simulink model "WormAndGearConstraint"  (R2024a)
settings: Solver=ode45  StartTime=0.0  StopTime=120  MaxStep=0.01  RelTol=1e-3
PreLoadFcn:
  | addpath(fullfile('WormAndGearConstraintSupport','Data'));
  | addpath(fullfile('WormAndGearConstraintSupport','Scripts'));
model workspace: external: MATLAB File WormAndGearConstraintParameters.m (data not in the file)
undefined symbols (not defined in the file or in its folder): slewdrive, X, Y, Z
libraries: sm_lib x75, neural x40, nesl_utility x38, fl_lib x32, WormAndGearConstraintLibrary x24, ee_lib x6, slpidlib x6, spsSeriesRLCBranchLib x2, fl_ps_legacy_lib x1, spsPWMGeneratorDCDCLib x1, spsMosfetLib x1, spsPVArrayLib x1
(part 6 of 6)

== system WormAndGearConstraint/Solar Array/Solar Tracker3/Slew Drive/Worm and Gear Assembly/Worm ==
  Left Non-Threaded : WormAndGearConstraintLibrary/Sliced Hollow Cylinder  outerRadius=wormNonThreadedRadius  thickness=wormNonThreadedThickness  length=wormNonThreadedLength  sliceThickness=wormSliceProportion*wormNonThreadedRadius  rho=wormRho  mainColor=wormColor  sliceColor=wormSliceColor
  Right Non-Threaded : WormAndGearConstraintLibrary/Sliced Hollow Cylinder  outerRadius=wormNonThreadedRadius  thickness=wormNonThreadedThickness  length=wormNonThreadedLength  sliceThickness=wormSliceProportion*wormNonThreadedRadius  rho=wormRho  mainColor=wormColor  sliceColor=wormSliceColor
  Threaded : WormAndGearConstraintLibrary/Sliced Hollow Cylinder  outerRadius=wormRadius  thickness=wormThreadedThickness  length=wormThreadedLength  sliceThickness=wormSliceProportion*wormRadius  rho=wormRho  mainColor=wormColor  sliceColor=wormSliceColor
  L : PMIOPort  Side=Left
  R : PMIOPort  Port=2  Side=Right
  connections:
  Threaded/LConn1 -- Left Non-Threaded/RConn1
  Threaded/RConn1 -- Right Non-Threaded/LConn1
  R/RConn1 -- Right Non-Threaded/RConn1
  Left Non-Threaded/LConn1 -- L/RConn1

== matlab function WormAndGearConstraint/Soalr Power Generation Calculation/Solar inputs1/MATLAB Function1 ==
  data: lat input; output output; lon input
function output = generateInput(lat, lon)
    % Get the current date and time
    datetimeNow = datetime('now');
    [~, month, day , hour, ~, ~] = datevec(datetimeNow);

    % Create the output array
    output = [lat; lon; month; day; hour];
end

== matlab function WormAndGearConstraint/Solar Array/MATLAB Function ==
  data: lat input; output output; lon input
function output = generateInput(lat, lon)
    % Get the current date and time
    datetimeNow = datetime('now');
    [~, month, day , hour, ~, ~] = datevec(datetimeNow);

    % Create the output array
    output = [lat; lon; month; day; hour];
end

== matlab function WormAndGearConstraint/MATLAB Function ==
  data latitude settings: description=Year input
  data: latitude input double size=1; azimuth output size=1; longitude input double size=1; timeVector input double size=[1 6]; elevation output double size=1
function [azimuth, elevation] = calculateSolarPosition(latitude, longitude, timeVector)
    year = timeVector(1);
    month = timeVector(2);
    day = timeVector(3);
    hour = timeVector(4);
    minute = timeVector(5);
    second = timeVector(6);

    % Calculate Julian Date
    JD = calculateJulianDate(year, month, day, hour, minute, second);
    
    % Calculate days since J2000.0
    n = daysSinceJ2000(JD);
    
    % Calculate mean longitude of the sun
    L = meanLongitudeSun(n);
    
    % Calculate mean anomaly of the sun
    g = meanAnomalySun(n);
    
    % Calculate ecliptic longitude of the sun
    lambda = eclipticLongitudeSun(L, g);
    
    % Calculate obliquity of the ecliptic
    epsilon = obliquityEcliptic(n);
    
    % Calculate right ascension and declination of the sun
    [alpha, delta] = rightAscensionDeclination(lambda, epsilon);
    
    % Calculate local sidereal time
    LST = localSiderealTime(n, longitude, hour, minute, second);
    
    % Calculate hour angle
    H = hourAngle(LST, alpha);
    
    % Calculate elevation and azimuth angles
    [elevation, azimuth] = solarElevationAzimuth(latitude, delta, H);
end

% Helper functions
function JD = calculateJulianDate(year, month, day, hour, minute, second)
    if month <= 2
        year = year - 1;
        month = month + 12;
    end
    A = floor(year / 100);
    B = 2 - A + floor(A / 4);
    JD = floor(365.25 * (year + 4716)) + floor(30.6001 * (month + 1)) + day + B - 1524.5 ...
        + (hour + minute / 60 + second / 3600) / 24;
end

function n = daysSinceJ2000(JD)
    JD_J2000 = 2451545.0;  % Julian Date of J2000.0
    n = JD - JD_J2000;
end

function L = meanLongitudeSun(n)
    L = mod(280.460 + 0.9856474 * n, 360);
end

function g = meanAnomalySun(n)
    g = mod(357.528 + 0.9856003 * n, 360);
end

function lambda = eclipticLongitudeSun(L, g)
    lambda = mod(L + 1.915 * sind(g) + 0.020 * sind(2 * g), 360);
end

function epsilon = obliquityEcliptic(n)
    epsilon = 23.439 - 0.0000004 * n;
end

function [alpha, delta] = rightAscensionDeclination(lambda, epsilon)
    alpha = atan2d(cosd(epsilon) * sind(lambda), cosd(lambda));
    delta = asind(sind(epsilon) * sind(lambda));
end

function LST = localSiderealTime(n, longitude, hour, minute, second)
    GMST = mod(6.697374558 + 0.06570982441908 * n + (hour + minute / 60 + second / 3600) * 1.00273790935, 24);
    LST = mod(GMST * 15 + longitude, 360);
end

function H = hourAngle(LST, alpha)
    H = mod(LST - alpha, 360);
end

function [elevation, azimuth] = solarElevationAzimuth(latitude, delta, H)
    elevation = asind(sind(latitude) * sind(delta) + cosd(latitude) * cosd(delta) * cosd(H));
    azimuth = atan2d(-sind(H), cosd(H) * sind(latitude) - tand(delta) * cosd(latitude));
    if azimuth < 0
        azimuth = azimuth + 360;
    end
end

== stateflow chart WormAndGearConstraint/Solar Array/stateflow logic chart ==
  state Night_time
    during:
    pitch_upd = 0 ;
    yaw_upd = 0 ;
  state Cloudy
    entry:
    hold_pitch = pitch ;
    hold_yaw  = yaw ;
    during :
    pitch_upd = hold_pitch
    yaw_upd = hold_yaw;
    exit:
    pitch_upd = hold_pitch
    yaw_upd = hold_yaw;
  state Daytime
    during :
    pitch_upd = pitch;
    yaw_upd = yaw;
  Cloudy -> Night_time [order 2] : [abs(pitch) > 1.48353]
  Night_time -> Cloudy [order 1] : [ irradiance <450 && abs(pitch)<=1.48353 ]
  Night_time -> Daytime [order 2] : [abs(pitch)<=1.48353]
  Daytime -> Night_time [order 1] : [abs(pitch) > 1.48353]
  (default) -> Daytime
  Daytime -> Cloudy [order 2] : [ irradiance < 450 ]
  Cloudy -> Daytime [order 1] : [abs(pitch)<=1.48353 && irradiance>= 450]
  data: yaw input; yaw_upd output; pitch input; pitch_upd output; hold_yaw local double size=1; hold_pitch local double size=1; irradiance input

== matlab function WormAndGearConstraint/MATLAB Function1 ==
  data: unused input double size=1; timeVector output double size=[1 6]
function timeVector = extractTimeFromClock(~)
    datetimeNow = datetime('now');
    [year, month, day, hour, minute, second] = datevec(datetimeNow);
    timeVector = [year, month, day, hour, minute, second];
end

== matlab function WormAndGearConstraint/Soalr Power Generation Calculation/Battery Energy Storage System/MATLAB Function ==
  data: currentSoC input; newSoC output; chargeCurrent input; dischargeCurrent input; batteryCapacity input; timeStep input
function newSoC = SoCCalculation(currentSoC, chargeCurrent, dischargeCurrent, batteryCapacity, timeStep)
    % Calculate the new state of charge
    newSoC = currentSoC + (chargeCurrent - dischargeCurrent) * timeStep / (batteryCapacity * 3600); % Convert capacity to Wh
    % Limit the SoC between 0 and 1
    newSoC = max(0, min(1, newSoC));
end

== matlab function WormAndGearConstraint/Soalr Power Generation Calculation/Battery Energy Storage System/MATLAB Function1 ==
  data: PVPower input; chargeCurrent output; LoadDemand input; SoC input
function chargeCurrent = chargeControl(PVPower, LoadDemand, SoC)
    maxChargeCurrent = 50; % Maximum charging current in amps
    batteryVoltage = 12; % Example battery voltage
    if SoC < 0.95 % Charge battery if SoC is less than 95%
        excessPower = PVPower - LoadDemand;
        chargeCurrent = min(excessPower / batteryVoltage, maxChargeCurrent); % Adjust based on battery voltage
    else
        chargeCurrent = 0; % Stop charging if SoC >= 95%
    end
end

== matlab function WormAndGearConstraint/Soalr Power Generation Calculation/Battery Energy Storage System/MATLAB Function2 ==
  data: PVPower input; dischargeCurrent output; LoadDemand input; SoC input
function dischargeCurrent = dischargeControl(PVPower, LoadDemand, SoC)
    maxDischargeCurrent = 50; % Maximum discharging current in amps
    batteryVoltage = 12; % Example battery voltage
    if SoC > 0.2 % Discharge battery if SoC is more than 20%
        deficitPower = LoadDemand - PVPower;
        dischargeCurrent = min(deficitPower / batteryVoltage, maxDischargeCurrent); % Adjust based on battery voltage
    else
        dischargeCurrent = 0; % Stop discharging if SoC <= 20%
    end
end

== matlab function WormAndGearConstraint/Soalr Power Generation Calculation/Optical model1/MATLAB Function ==
  data: S2 input; Ir2 output; Incl input
function Ir2 = optics2(S2, Incl)
    
    %This function computes the reflection, absorption and transmission in
    %the glass to compute the irradiation to the PV cells, the heat absorbed 
    %in the glass and the radiation power absorbed in the PV cells,
    %it is based on Fresnel's laws, depending on the incident angle
    
    Ncell =  72;
    Acell =  0.0225;
    ng = 1.52;
    absg = 0.2;
    dg = 0.01;
    rpv = 0.15;
   

    % Fresnel equations 1st boundary
    r1p =  ( ng^2*cos(Incl) - sqrt(ng^2 - sin(Incl)^2) )^2/( ng^2*cos(Incl) + sqrt( ng^2 - sin(Incl)^2 ) )^2; %P polarization
    r1s =  ( cos(Incl) - sqrt(ng^2 - sin(Incl)^2) )^2/( cos(Incl) + sqrt( ng^2 - sin(Incl)^2 ) )^2; %S polarization
    r1 = 0.5*(r1p + r1s); %Effective reflectance
    t1 = 1-r1;

    nga = 1/ng; %refractive index glass -> air
    th2 = asin(sin(Incl)/ng);  %Snell's law to compute angle of incidence on 2nd boundary

    % Fresnel equations 2nd boundary
    r2p = ( nga^2*cos(th2) - sqrt(nga^2 - sin(th2)^2) )^2/( nga^2*cos(th2) + sqrt( nga^2 - sin(th2)^2 ) )^2 ;
    r2s = ( cos(th2) - sqrt(nga^2 - sin(th2)^2) )^2/( cos(th2) + sqrt( nga^2 - sin(th2)^2 ) )^2 ;
    r2 = 0.5*(r2p + r2s); %Effective reflectance
    t2 = 1 - r2;

    taug = exp(-absg*dg/cos(th2)); 
    
    %Total coefficients for infinite reflections between 2 parallel boundaries
    Transg = t1*taug*t2/(1 - r1*r2*taug^2);
    Reflg = r1 + (t1^2*taug^2*r2)/(1 - r1*r2*taug^2);
    Absg = 1 - Transg - Reflg; 

    Ir2 = S2*Transg; %Irradiation to the PV cells
    heatg = Acell*Ncell*Absg*S2; %heat absorbed in the glass
    powAbspv = Acell*Ncell*Transg*(1-rpv)*S2; %radiation power absorbed by PV cells. Part of it transforms in electrical power
    
end
